simulink model "Quad_Nonlinear_Roll_Model"  (R2020a)
settings: Solver=ode4  StartTime=0.0  StopTime=0.5  FixedStep=0.01  RelTol=1e-3
values from neighbouring files (symbols this model uses):
  A1 = (h_cg * g * m_tot) / (m_tot * h_cg^2 + J_xx)    [QuadConstants.m]    (also in roll_parameter_estiation_result_I.m = 4.15251143915)
  A3 = (b * d_cg) / (m_tot * h_cg^2 + J_xx)    [QuadConstants.m]
  A5 = (m1 * g * miu_k * r_x) / (m_tot * h_cg^2 + J_xx)    [QuadConstants.m]    (also in roll_parameter_estiation_result_I.m = -0.190519012325)
  A6 = 0    [QuadConstants.m]    (also in roll_parameter_estiation_result_I.m = 0.650604724883)
  init_I = data_I(1, :)    [load_data.m]
  init_II = data_II(1, :)    [load_data.m]
  init_III = data_III(1, :)    [load_data.m]
  init_IV = data_IV(1, :)    [load_data.m]
undefined symbols (not defined in the file or in its folder): init_V, magnitude
settings Model: OrderedModelArguments=off  Creator=Ali  LastModifiedBy=Ali

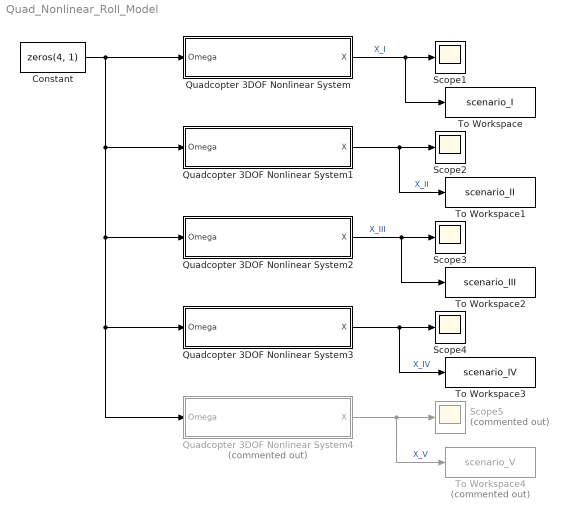
== system Quad_Nonlinear_Roll_Model ==
  Constant : Constant  Value=zeros(4, 1)
  Quadcopter 3DOF Nonlinear System : Subsystem  TreatAsAtomicUnit=on
  Quadcopter 3DOF Nonlinear System1 : Subsystem  TreatAsAtomicUnit=on
  Quadcopter 3DOF Nonlinear System2 : Subsystem  TreatAsAtomicUnit=on
  Quadcopter 3DOF Nonlinear System3 : Subsystem  TreatAsAtomicUnit=on
  Quadcopter 3DOF Nonlinear System4 : Subsystem  Commented=on  TreatAsAtomicUnit=on
  Scope{1..4} (4 alike) : Scope
  Scope5 : Scope  Commented=on
  To Workspace : ToWorkspace  VariableName=scenario_I  SampleTime=-1
  To Workspace1 : ToWorkspace  VariableName=scenario_II  SampleTime=-1
  To Workspace2 : ToWorkspace  VariableName=scenario_III  SampleTime=-1
  To Workspace3 : ToWorkspace  VariableName=scenario_IV  SampleTime=-1
  To Workspace4 : ToWorkspace  Commented=on  VariableName=scenario_V  SampleTime=-1
  wires:
  Constant/1 -> Quadcopter 3DOF Nonlinear System/1(Omega), Quadcopter 3DOF Nonlinear System4/1(Omega), Quadcopter 3DOF Nonlinear System3/1(Omega), Quadcopter 3DOF Nonlinear System2/1(Omega), Quadcopter 3DOF Nonlinear System1/1(Omega)
  Quadcopter 3DOF Nonlinear System1/1(X) -> To Workspace1/1, Scope2/1  "X_II"
  Quadcopter 3DOF Nonlinear System/1(X) -> To Workspace/1, Scope1/1  "X_I"
  Quadcopter 3DOF Nonlinear System2/1(X) -> To Workspace2/1, Scope3/1  "X_III"
  Quadcopter 3DOF Nonlinear System3/1(X) -> To Workspace3/1, Scope4/1  "X_IV"
  Quadcopter 3DOF Nonlinear System4/1(X) -> To Workspace4/1, Scope5/1  "X_V"

== system Quad_Nonlinear_Roll_Model/Quadcopter 3DOF Nonlinear System ==
  Omega : Inport
  Integrator : Integrator  InitialCondition=init_I
  Quad System : Subsystem
  X : Outport
  wires:
  Integrator/1 -> Quad System/1(X), X/1  "X"
  Quad System/1(dot(X)) -> Integrator/1  "dot(X)"
  Omega/1 -> Quad System/2(Omega)

== system Quad_Nonlinear_Roll_Model/Quadcopter 3DOF Nonlinear System1 ==
  Omega : Inport
  Integrator : Integrator  InitialCondition=init_II
  Quad System : Subsystem
  X : Outport
  wires:
  Integrator/1 -> Quad System/1(X), X/1  "X"
  Quad System/1(dot(X)) -> Integrator/1  "dot(X)"
  Omega/1 -> Quad System/2(Omega)

== system Quad_Nonlinear_Roll_Model/Quadcopter 3DOF Nonlinear System2 ==
  Omega : Inport
  Integrator : Integrator  InitialCondition=init_III
  Quad System : Subsystem
  X : Outport
  wires:
  Integrator/1 -> Quad System/1(X), X/1  "X"
  Quad System/1(dot(X)) -> Integrator/1  "dot(X)"
  Omega/1 -> Quad System/2(Omega)

== system Quad_Nonlinear_Roll_Model/Quadcopter 3DOF Nonlinear System3 ==
  Omega : Inport
  Integrator : Integrator  InitialCondition=init_IV
  Quad System : Subsystem
  X : Outport
  wires:
  Integrator/1 -> Quad System/1(X), X/1  "X"
  Quad System/1(dot(X)) -> Integrator/1  "dot(X)"
  Omega/1 -> Quad System/2(Omega)

== system Quad_Nonlinear_Roll_Model/Quadcopter 3DOF Nonlinear System4 ==
  Omega : Inport
  Integrator : Integrator  InitialCondition=init_V
  Quad System : Subsystem
  X : Outport
  wires:
  Integrator/1 -> Quad System/1(X), X/1  "X"
  Quad System/1(dot(X)) -> Integrator/1  "dot(X)"
  Omega/1 -> Quad System/2(Omega)

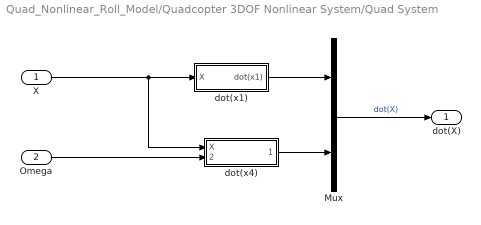
== system Quad_Nonlinear_Roll_Model/Quadcopter 3DOF Nonlinear System/Quad System ==
  X : Inport
  Omega : Inport  Port=2
  Mux : Mux  Inputs=2
  dot(x1) : Subsystem
  dot(x4) : Subsystem
  dot(X) : Outport
  wires:
  Mux/1 -> dot(X)/1  "dot(X)"
  X/1 -> dot(x4)/1(X), dot(x1)/1(X)
  Omega/1 -> dot(x4)/2(Omega)
  dot(x1)/1(dot(x1)) -> Mux/1
  dot(x4)/1(dot(x4)) -> Mux/2

== system Quad_Nonlinear_Roll_Model/Quadcopter 3DOF Nonlinear System1/Quad System ==
  X : Inport
  Omega : Inport  Port=2
  Mux : Mux  Inputs=2
  dot(x1) : Subsystem
  dot(x4) : Subsystem
  dot(X) : Outport
  wires:
  Mux/1 -> dot(X)/1  "dot(X)"
  X/1 -> dot(x4)/1(X), dot(x1)/1(X)
  Omega/1 -> dot(x4)/2(Omega)
  dot(x1)/1(dot(x1)) -> Mux/1
  dot(x4)/1(dot(x4)) -> Mux/2

== system Quad_Nonlinear_Roll_Model/Quadcopter 3DOF Nonlinear System2/Quad System ==
  X : Inport
  Omega : Inport  Port=2
  Mux : Mux  Inputs=2
  dot(x1) : Subsystem
  dot(x4) : Subsystem
  dot(X) : Outport
  wires:
  Mux/1 -> dot(X)/1  "dot(X)"
  X/1 -> dot(x4)/1(X), dot(x1)/1(X)
  Omega/1 -> dot(x4)/2(Omega)
  dot(x1)/1(dot(x1)) -> Mux/1
  dot(x4)/1(dot(x4)) -> Mux/2

== system Quad_Nonlinear_Roll_Model/Quadcopter 3DOF Nonlinear System3/Quad System ==
  X : Inport
  Omega : Inport  Port=2
  Mux : Mux  Inputs=2
  dot(x1) : Subsystem
  dot(x4) : Subsystem
  dot(X) : Outport
  wires:
  Mux/1 -> dot(X)/1  "dot(X)"
  X/1 -> dot(x4)/1(X), dot(x1)/1(X)
  Omega/1 -> dot(x4)/2(Omega)
  dot(x1)/1(dot(x1)) -> Mux/1
  dot(x4)/1(dot(x4)) -> Mux/2

== system Quad_Nonlinear_Roll_Model/Quadcopter 3DOF Nonlinear System4/Quad System ==
  X : Inport
  Omega : Inport  Port=2
  Mux : Mux  Inputs=2
  dot(x1) : Subsystem
  dot(x4) : Subsystem
  dot(X) : Outport
  wires:
  Mux/1 -> dot(X)/1  "dot(X)"
  X/1 -> dot(x4)/1(X), dot(x1)/1(X)
  Omega/1 -> dot(x4)/2(Omega)
  dot(x1)/1(dot(x1)) -> Mux/1
  dot(x4)/1(dot(x4)) -> Mux/2

== system Quad_Nonlinear_Roll_Model/Quadcopter 3DOF Nonlinear System/Quad System/dot(x1) ==
  X : Inport
  Subsystem1 : Subsystem
  dot(x1) : Outport
  wires:
  X/1 -> Subsystem1/1(X)  "X"
  Subsystem1/1(x4) -> dot(x1)/1

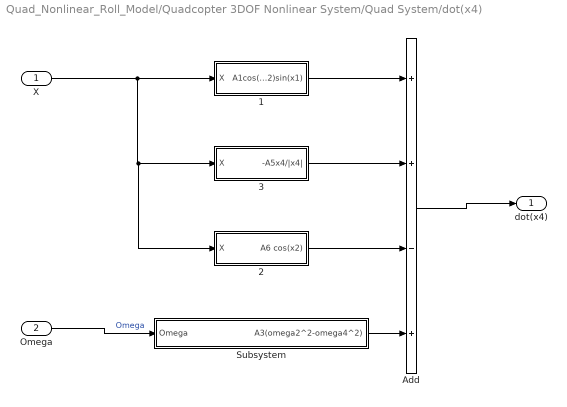
== system Quad_Nonlinear_Roll_Model/Quadcopter 3DOF Nonlinear System/Quad System/dot(x4) ==
  X : Inport
  Omega : Inport  Port=2
  1 : Subsystem
  2 : Subsystem
  3 : Subsystem
  Add : Sum  Inputs=++-+
  Subsystem : Subsystem
  dot(x4) : Outport
  wires:
  Omega/1 -> Subsystem/1(Omega)  "Omega"
  Add/1 -> dot(x4)/1
  1/1(A1cos(x2)sin(x1)) -> Add/1
  3/1("-A5x4/|x4| ") -> Add/2
  X/1 -> 2/1(X), 3/1(X), 1/1(X)
  2/1(A6 cos(x2)) -> Add/3
  Subsystem/1(A3(omega2^2-omega4^2)) -> Add/4

== system Quad_Nonlinear_Roll_Model/Quadcopter 3DOF Nonlinear System1/Quad System/dot(x1) ==
  X : Inport
  Subsystem1 : Subsystem
  dot(x1) : Outport
  wires:
  X/1 -> Subsystem1/1(X)  "X"
  Subsystem1/1(x4) -> dot(x1)/1

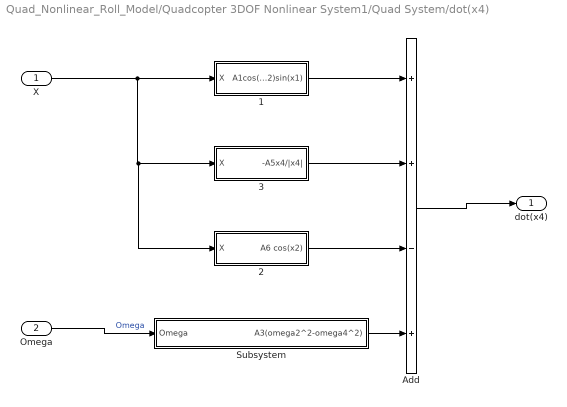
== system Quad_Nonlinear_Roll_Model/Quadcopter 3DOF Nonlinear System1/Quad System/dot(x4) ==
  X : Inport
  Omega : Inport  Port=2
  1 : Subsystem
  2 : Subsystem
  3 : Subsystem
  Add : Sum  Inputs=++-+
  Subsystem : Subsystem
  dot(x4) : Outport
  wires:
  Omega/1 -> Subsystem/1(Omega)  "Omega"
  Add/1 -> dot(x4)/1
  1/1(A1cos(x2)sin(x1)) -> Add/1
  3/1("-A5x4/|x4| ") -> Add/2
  X/1 -> 2/1(X), 3/1(X), 1/1(X)
  2/1(A6 cos(x2)) -> Add/3
  Subsystem/1(A3(omega2^2-omega4^2)) -> Add/4

== system Quad_Nonlinear_Roll_Model/Quadcopter 3DOF Nonlinear System2/Quad System/dot(x1) ==
  X : Inport
  Subsystem1 : Subsystem
  dot(x1) : Outport
  wires:
  X/1 -> Subsystem1/1(X)  "X"
  Subsystem1/1(x4) -> dot(x1)/1

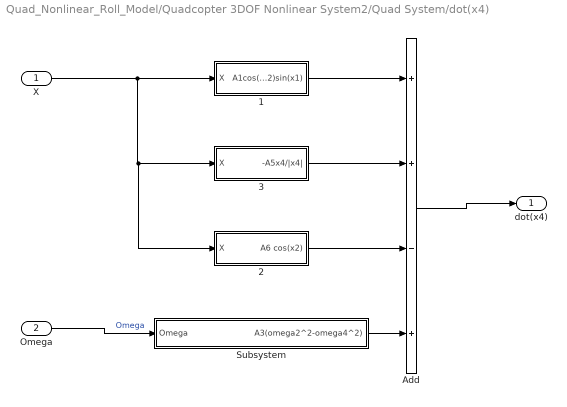
== system Quad_Nonlinear_Roll_Model/Quadcopter 3DOF Nonlinear System2/Quad System/dot(x4) ==
  X : Inport
  Omega : Inport  Port=2
  1 : Subsystem
  2 : Subsystem
  3 : Subsystem
  Add : Sum  Inputs=++-+
  Subsystem : Subsystem
  dot(x4) : Outport
  wires:
  Omega/1 -> Subsystem/1(Omega)  "Omega"
  Add/1 -> dot(x4)/1
  1/1(A1cos(x2)sin(x1)) -> Add/1
  3/1("-A5x4/|x4| ") -> Add/2
  X/1 -> 2/1(X), 3/1(X), 1/1(X)
  2/1(A6 cos(x2)) -> Add/3
  Subsystem/1(A3(omega2^2-omega4^2)) -> Add/4

== system Quad_Nonlinear_Roll_Model/Quadcopter 3DOF Nonlinear System3/Quad System/dot(x1) ==
  X : Inport
  Subsystem1 : Subsystem
  dot(x1) : Outport
  wires:
  X/1 -> Subsystem1/1(X)  "X"
  Subsystem1/1(x4) -> dot(x1)/1

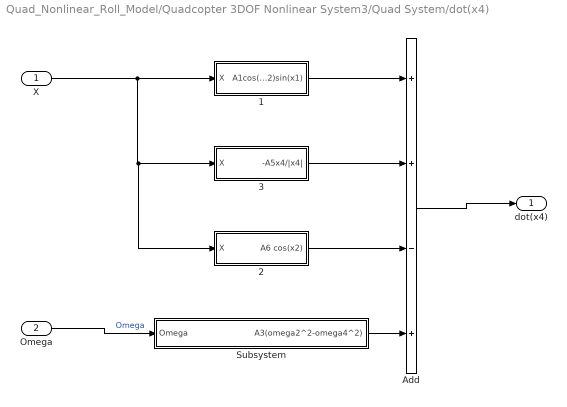
== system Quad_Nonlinear_Roll_Model/Quadcopter 3DOF Nonlinear System3/Quad System/dot(x4) ==
  X : Inport
  Omega : Inport  Port=2
  1 : Subsystem
  2 : Subsystem
  3 : Subsystem
  Add : Sum  Inputs=++-+
  Subsystem : Subsystem
  dot(x4) : Outport
  wires:
  Omega/1 -> Subsystem/1(Omega)  "Omega"
  Add/1 -> dot(x4)/1
  1/1(A1cos(x2)sin(x1)) -> Add/1
  3/1("-A5x4/|x4| ") -> Add/2
  X/1 -> 2/1(X), 3/1(X), 1/1(X)
  2/1(A6 cos(x2)) -> Add/3
  Subsystem/1(A3(omega2^2-omega4^2)) -> Add/4

== system Quad_Nonlinear_Roll_Model/Quadcopter 3DOF Nonlinear System4/Quad System/dot(x1) ==
  X : Inport
  Subsystem1 : Subsystem
  dot(x1) : Outport
  wires:
  X/1 -> Subsystem1/1(X)  "X"
  Subsystem1/1(x4) -> dot(x1)/1

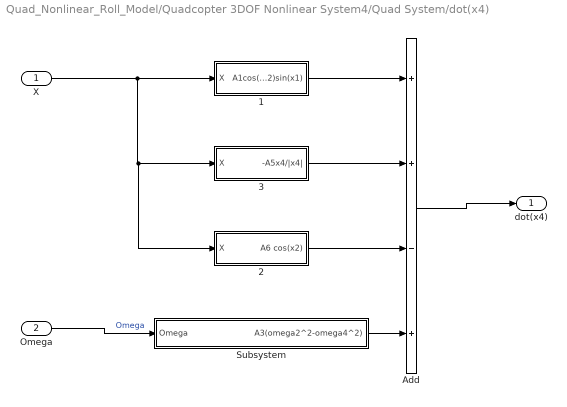
== system Quad_Nonlinear_Roll_Model/Quadcopter 3DOF Nonlinear System4/Quad System/dot(x4) ==
  X : Inport
  Omega : Inport  Port=2
  1 : Subsystem
  2 : Subsystem
  3 : Subsystem
  Add : Sum  Inputs=++-+
  Subsystem : Subsystem
  dot(x4) : Outport
  wires:
  Omega/1 -> Subsystem/1(Omega)  "Omega"
  Add/1 -> dot(x4)/1
  1/1(A1cos(x2)sin(x1)) -> Add/1
  3/1("-A5x4/|x4| ") -> Add/2
  X/1 -> 2/1(X), 3/1(X), 1/1(X)
  2/1(A6 cos(x2)) -> Add/3
  Subsystem/1(A3(omega2^2-omega4^2)) -> Add/4

== system Quad_Nonlinear_Roll_Model/Quadcopter 3DOF Nonlinear System/Quad System/dot(x1)/Subsystem1 ==
  X : Inport
  Selector : Selector  InputPortWidth=2  IndexOptions=Index vector (dialog)  Indices=[2]  OutputSizes=1
  x4 : Outport
  wires:
  Selector/1 -> x4/1
  X/1 -> Selector/1

== system Quad_Nonlinear_Roll_Model/Quadcopter 3DOF Nonlinear System/Quad System/dot(x4)/1 ==
  X : Inport
  Selector : Selector  InputPortWidth=2  IndexOptions=Index vector (dialog)  Indices=[1]  OutputSizes=1
  Subsystem : Subsystem
  A1cos(x2)sin(x1) : Outport
  wires:
  Selector/1 -> Subsystem/1(x1)  "x1"
  Subsystem/1(A1cos(x2)sin(x1)) -> A1cos(x2)sin(x1)/1
  X/1 -> Selector/1  "x"

== system Quad_Nonlinear_Roll_Model/Quadcopter 3DOF Nonlinear System/Quad System/dot(x4)/2 ==
  X : Inport
  Selector : Selector  InputPortWidth=2  IndexOptions=Index vector (dialog)  Indices=[1]  OutputSizes=1
  Subsystem : Subsystem
  A6 cos(x2) : Outport
  wires:
  X/1 -> Selector/1  "x"
  Subsystem/1(A6 cos(x1)) -> A6 cos(x2)/1
  Selector/1 -> Subsystem/1(x1)

== system Quad_Nonlinear_Roll_Model/Quadcopter 3DOF Nonlinear System/Quad System/dot(x4)/3 ==
  X : Inport
  Selector : Selector  InputPortWidth=2  IndexOptions=Index vector (dialog)  Indices=[2]  OutputSizes=1
  Subsystem : Subsystem
  "-A5x4/|x4| " : Outport
  wires:
  Subsystem/1("-A5x4/|x4| ") -> "-A5x4/|x4| "/1
  X/1 -> Selector/1  "x"
  Selector/1 -> Subsystem/1(x4)

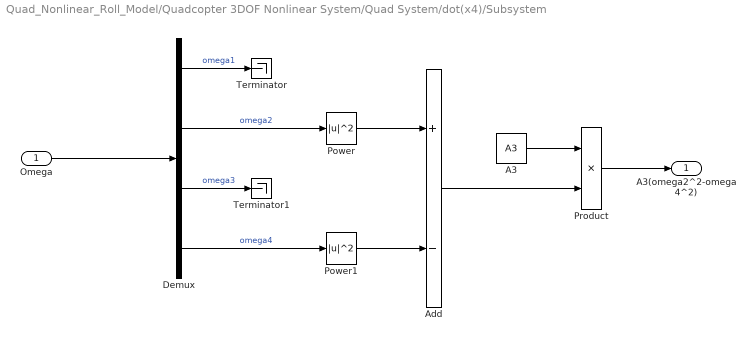
== system Quad_Nonlinear_Roll_Model/Quadcopter 3DOF Nonlinear System/Quad System/dot(x4)/Subsystem ==
  Omega : Inport
  A3 : Constant  Value=A3
  Add : Sum  Inputs=+-
  Demux : Demux
  Power : Math  Operator=magnitude^2  SaturateOnIntegerOverflow=on
  Power1 : Math  Operator=magnitude^2  SaturateOnIntegerOverflow=on
  Product : Product
  Terminator : Terminator
  Terminator1 : Terminator
  A3(omega2^2-omega4^2) : Outport
  wires:
  Product/1 -> A3(omega2^2-omega4^2)/1
  Power1/1 -> Add/2
  Demux/2 -> Power/1  "omega2"
  Demux/4 -> Power1/1  "omega4"
  Add/1 -> Product/2
  Power/1 -> Add/1
  A3/1 -> Product/1
  Omega/1 -> Demux/1
  Demux/3 -> Terminator1/1  "omega3"
  Demux/1 -> Terminator/1  "omega1"

== system Quad_Nonlinear_Roll_Model/Quadcopter 3DOF Nonlinear System1/Quad System/dot(x1)/Subsystem1 ==
  X : Inport
  Selector : Selector  InputPortWidth=2  IndexOptions=Index vector (dialog)  Indices=[2]  OutputSizes=1
  x4 : Outport
  wires:
  Selector/1 -> x4/1
  X/1 -> Selector/1

== system Quad_Nonlinear_Roll_Model/Quadcopter 3DOF Nonlinear System1/Quad System/dot(x4)/1 ==
  X : Inport
  Selector : Selector  InputPortWidth=2  IndexOptions=Index vector (dialog)  Indices=[1]  OutputSizes=1
  Subsystem : Subsystem
  A1cos(x2)sin(x1) : Outport
  wires:
  Selector/1 -> Subsystem/1(x1)  "x1"
  Subsystem/1(A1cos(x2)sin(x1)) -> A1cos(x2)sin(x1)/1
  X/1 -> Selector/1  "x"

== system Quad_Nonlinear_Roll_Model/Quadcopter 3DOF Nonlinear System1/Quad System/dot(x4)/2 ==
  X : Inport
  Selector : Selector  InputPortWidth=2  IndexOptions=Index vector (dialog)  Indices=[1]  OutputSizes=1
  Subsystem : Subsystem
  A6 cos(x2) : Outport
  wires:
  X/1 -> Selector/1  "x"
  Subsystem/1(A6 cos(x1)) -> A6 cos(x2)/1
  Selector/1 -> Subsystem/1(x1)

== system Quad_Nonlinear_Roll_Model/Quadcopter 3DOF Nonlinear System1/Quad System/dot(x4)/3 ==
  X : Inport
  Selector : Selector  InputPortWidth=2  IndexOptions=Index vector (dialog)  Indices=[2]  OutputSizes=1
  Subsystem : Subsystem
  "-A5x4/|x4| " : Outport
  wires:
  Subsystem/1("-A5x4/|x4| ") -> "-A5x4/|x4| "/1
  X/1 -> Selector/1  "x"
  Selector/1 -> Subsystem/1(x4)

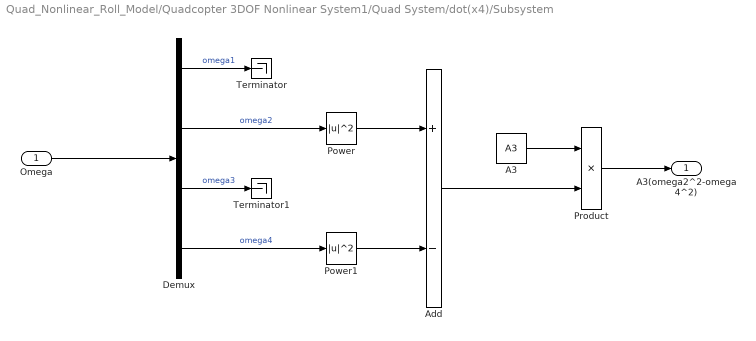
== system Quad_Nonlinear_Roll_Model/Quadcopter 3DOF Nonlinear System1/Quad System/dot(x4)/Subsystem ==
  Omega : Inport
  A3 : Constant  Value=A3
  Add : Sum  Inputs=+-
  Demux : Demux
  Power : Math  Operator=magnitude^2  SaturateOnIntegerOverflow=on
  Power1 : Math  Operator=magnitude^2  SaturateOnIntegerOverflow=on
  Product : Product
  Terminator : Terminator
  Terminator1 : Terminator
  A3(omega2^2-omega4^2) : Outport
  wires:
  Product/1 -> A3(omega2^2-omega4^2)/1
  Power1/1 -> Add/2
  Demux/2 -> Power/1  "omega2"
  Demux/4 -> Power1/1  "omega4"
  Add/1 -> Product/2
  Power/1 -> Add/1
  A3/1 -> Product/1
  Omega/1 -> Demux/1
  Demux/3 -> Terminator1/1  "omega3"
  Demux/1 -> Terminator/1  "omega1"

== system Quad_Nonlinear_Roll_Model/Quadcopter 3DOF Nonlinear System2/Quad System/dot(x1)/Subsystem1 ==
  X : Inport
  Selector : Selector  InputPortWidth=2  IndexOptions=Index vector (dialog)  Indices=[2]  OutputSizes=1
  x4 : Outport
  wires:
  Selector/1 -> x4/1
  X/1 -> Selector/1

== system Quad_Nonlinear_Roll_Model/Quadcopter 3DOF Nonlinear System2/Quad System/dot(x4)/1 ==
  X : Inport
  Selector : Selector  InputPortWidth=2  IndexOptions=Index vector (dialog)  Indices=[1]  OutputSizes=1
  Subsystem : Subsystem
  A1cos(x2)sin(x1) : Outport
  wires:
  Selector/1 -> Subsystem/1(x1)  "x1"
  Subsystem/1(A1cos(x2)sin(x1)) -> A1cos(x2)sin(x1)/1
  X/1 -> Selector/1  "x"

== system Quad_Nonlinear_Roll_Model/Quadcopter 3DOF Nonlinear System2/Quad System/dot(x4)/2 ==
  X : Inport
  Selector : Selector  InputPortWidth=2  IndexOptions=Index vector (dialog)  Indices=[1]  OutputSizes=1
  Subsystem : Subsystem
  A6 cos(x2) : Outport
  wires:
  X/1 -> Selector/1  "x"
  Subsystem/1(A6 cos(x1)) -> A6 cos(x2)/1
  Selector/1 -> Subsystem/1(x1)

== system Quad_Nonlinear_Roll_Model/Quadcopter 3DOF Nonlinear System2/Quad System/dot(x4)/3 ==
  X : Inport
  Selector : Selector  InputPortWidth=2  IndexOptions=Index vector (dialog)  Indices=[2]  OutputSizes=1
  Subsystem : Subsystem
  "-A5x4/|x4| " : Outport
  wires:
  Subsystem/1("-A5x4/|x4| ") -> "-A5x4/|x4| "/1
  X/1 -> Selector/1  "x"
  Selector/1 -> Subsystem/1(x4)

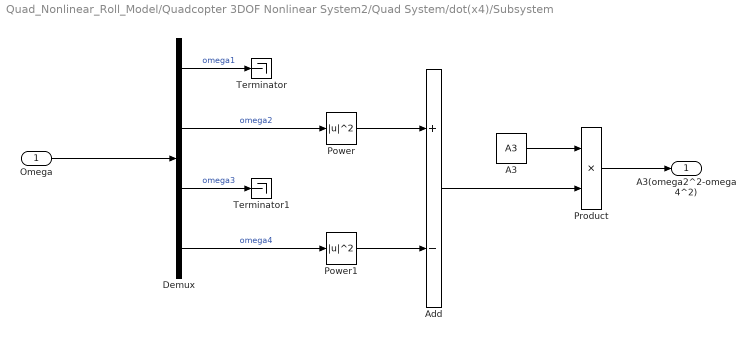
== system Quad_Nonlinear_Roll_Model/Quadcopter 3DOF Nonlinear System2/Quad System/dot(x4)/Subsystem ==
  Omega : Inport
  A3 : Constant  Value=A3
  Add : Sum  Inputs=+-
  Demux : Demux
  Power : Math  Operator=magnitude^2  SaturateOnIntegerOverflow=on
  Power1 : Math  Operator=magnitude^2  SaturateOnIntegerOverflow=on
  Product : Product
  Terminator : Terminator
  Terminator1 : Terminator
  A3(omega2^2-omega4^2) : Outport
  wires:
  Product/1 -> A3(omega2^2-omega4^2)/1
  Power1/1 -> Add/2
  Demux/2 -> Power/1  "omega2"
  Demux/4 -> Power1/1  "omega4"
  Add/1 -> Product/2
  Power/1 -> Add/1
  A3/1 -> Product/1
  Omega/1 -> Demux/1
  Demux/3 -> Terminator1/1  "omega3"
  Demux/1 -> Terminator/1  "omega1"

== system Quad_Nonlinear_Roll_Model/Quadcopter 3DOF Nonlinear System3/Quad System/dot(x1)/Subsystem1 ==
  X : Inport
  Selector : Selector  InputPortWidth=2  IndexOptions=Index vector (dialog)  Indices=[2]  OutputSizes=1
  x4 : Outport
  wires:
  Selector/1 -> x4/1
  X/1 -> Selector/1

== system Quad_Nonlinear_Roll_Model/Quadcopter 3DOF Nonlinear System3/Quad System/dot(x4)/1 ==
  X : Inport
  Selector : Selector  InputPortWidth=2  IndexOptions=Index vector (dialog)  Indices=[1]  OutputSizes=1
  Subsystem : Subsystem
  A1cos(x2)sin(x1) : Outport
  wires:
  Selector/1 -> Subsystem/1(x1)  "x1"
  Subsystem/1(A1cos(x2)sin(x1)) -> A1cos(x2)sin(x1)/1
  X/1 -> Selector/1  "x"

== system Quad_Nonlinear_Roll_Model/Quadcopter 3DOF Nonlinear System3/Quad System/dot(x4)/2 ==
  X : Inport
  Selector : Selector  InputPortWidth=2  IndexOptions=Index vector (dialog)  Indices=[1]  OutputSizes=1
  Subsystem : Subsystem
  A6 cos(x2) : Outport
  wires:
  X/1 -> Selector/1  "x"
  Subsystem/1(A6 cos(x1)) -> A6 cos(x2)/1
  Selector/1 -> Subsystem/1(x1)

== system Quad_Nonlinear_Roll_Model/Quadcopter 3DOF Nonlinear System3/Quad System/dot(x4)/3 ==
  X : Inport
  Selector : Selector  InputPortWidth=2  IndexOptions=Index vector (dialog)  Indices=[2]  OutputSizes=1
  Subsystem : Subsystem
  "-A5x4/|x4| " : Outport
  wires:
  Subsystem/1("-A5x4/|x4| ") -> "-A5x4/|x4| "/1
  X/1 -> Selector/1  "x"
  Selector/1 -> Subsystem/1(x4)

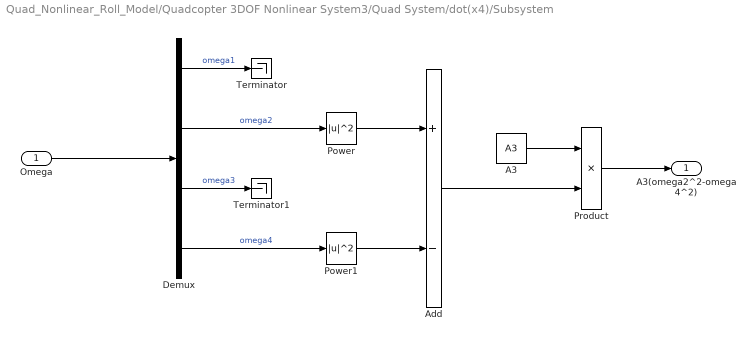
== system Quad_Nonlinear_Roll_Model/Quadcopter 3DOF Nonlinear System3/Quad System/dot(x4)/Subsystem ==
  Omega : Inport
  A3 : Constant  Value=A3
  Add : Sum  Inputs=+-
  Demux : Demux
  Power : Math  Operator=magnitude^2  SaturateOnIntegerOverflow=on
  Power1 : Math  Operator=magnitude^2  SaturateOnIntegerOverflow=on
  Product : Product
  Terminator : Terminator
  Terminator1 : Terminator
  A3(omega2^2-omega4^2) : Outport
  wires:
  Product/1 -> A3(omega2^2-omega4^2)/1
  Power1/1 -> Add/2
  Demux/2 -> Power/1  "omega2"
  Demux/4 -> Power1/1  "omega4"
  Add/1 -> Product/2
  Power/1 -> Add/1
  A3/1 -> Product/1
  Omega/1 -> Demux/1
  Demux/3 -> Terminator1/1  "omega3"
  Demux/1 -> Terminator/1  "omega1"

== system Quad_Nonlinear_Roll_Model/Quadcopter 3DOF Nonlinear System4/Quad System/dot(x1)/Subsystem1 ==
  X : Inport
  Selector : Selector  InputPortWidth=2  IndexOptions=Index vector (dialog)  Indices=[2]  OutputSizes=1
  x4 : Outport
  wires:
  Selector/1 -> x4/1
  X/1 -> Selector/1

== system Quad_Nonlinear_Roll_Model/Quadcopter 3DOF Nonlinear System4/Quad System/dot(x4)/1 ==
  X : Inport
  Selector : Selector  InputPortWidth=2  IndexOptions=Index vector (dialog)  Indices=[1]  OutputSizes=1
  Subsystem : Subsystem
  A1cos(x2)sin(x1) : Outport
  wires:
  Selector/1 -> Subsystem/1(x1)  "x1"
  Subsystem/1(A1cos(x2)sin(x1)) -> A1cos(x2)sin(x1)/1
  X/1 -> Selector/1  "x"

== system Quad_Nonlinear_Roll_Model/Quadcopter 3DOF Nonlinear System4/Quad System/dot(x4)/2 ==
  X : Inport
  Selector : Selector  InputPortWidth=2  IndexOptions=Index vector (dialog)  Indices=[1]  OutputSizes=1
  Subsystem : Subsystem
  A6 cos(x2) : Outport
  wires:
  X/1 -> Selector/1  "x"
  Subsystem/1(A6 cos(x1)) -> A6 cos(x2)/1
  Selector/1 -> Subsystem/1(x1)

== system Quad_Nonlinear_Roll_Model/Quadcopter 3DOF Nonlinear System4/Quad System/dot(x4)/3 ==
  X : Inport
  Selector : Selector  InputPortWidth=2  IndexOptions=Index vector (dialog)  Indices=[2]  OutputSizes=1
  Subsystem : Subsystem
  "-A5x4/|x4| " : Outport
  wires:
  Subsystem/1("-A5x4/|x4| ") -> "-A5x4/|x4| "/1
  X/1 -> Selector/1  "x"
  Selector/1 -> Subsystem/1(x4)

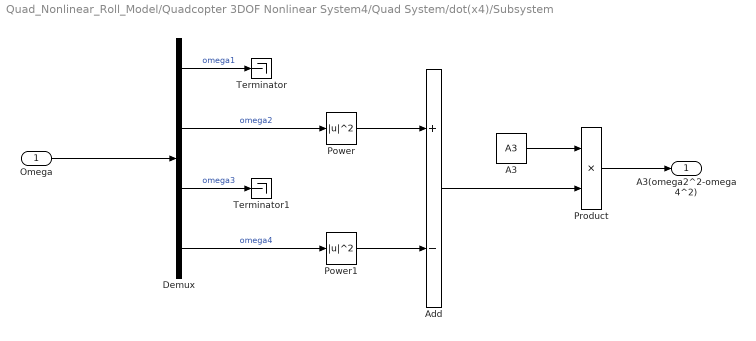
== system Quad_Nonlinear_Roll_Model/Quadcopter 3DOF Nonlinear System4/Quad System/dot(x4)/Subsystem ==
  Omega : Inport
  A3 : Constant  Value=A3
  Add : Sum  Inputs=+-
  Demux : Demux
  Power : Math  Operator=magnitude^2  SaturateOnIntegerOverflow=on
  Power1 : Math  Operator=magnitude^2  SaturateOnIntegerOverflow=on
  Product : Product
  Terminator : Terminator
  Terminator1 : Terminator
  A3(omega2^2-omega4^2) : Outport
  wires:
  Product/1 -> A3(omega2^2-omega4^2)/1
  Power1/1 -> Add/2
  Demux/2 -> Power/1  "omega2"
  Demux/4 -> Power1/1  "omega4"
  Add/1 -> Product/2
  Power/1 -> Add/1
  A3/1 -> Product/1
  Omega/1 -> Demux/1
  Demux/3 -> Terminator1/1  "omega3"
  Demux/1 -> Terminator/1  "omega1"

== system Quad_Nonlinear_Roll_Model/Quadcopter 3DOF Nonlinear System/Quad System/dot(x4)/1/Subsystem ==
  x1 : Inport
  A1 : Constant  Value=A1
  Product : Product
  Sin : Trigonometry
  A1cos(x2)sin(x1) : Outport
  wires:
  Sin/1 -> Product/1
  Product/1 -> A1cos(x2)sin(x1)/1
  x1/1 -> Sin/1
  A1/1 -> Product/2

== system Quad_Nonlinear_Roll_Model/Quadcopter 3DOF Nonlinear System/Quad System/dot(x4)/2/Subsystem ==
  x1 : Inport
  A6 : Constant  Value=A6
  Cos : Trigonometry  Operator=cos
  Product : Product
  A6 cos(x1) : Outport
  wires:
  A6/1 -> Product/1
  Product/1 -> A6 cos(x1)/1
  x1/1 -> Cos/1
  Cos/1 -> Product/2

== system Quad_Nonlinear_Roll_Model/Quadcopter 3DOF Nonlinear System/Quad System/dot(x4)/3/Subsystem ==
  x4 : Inport
  A5 : Constant  Value=A5
  Gain : Gain  Gain=-1
  Switch : Switch  Criteria=u2 > Threshold
  "-A5x4/|x4| " : Outport
  wires:
  Switch/1 -> "-A5x4/|x4| "/1
  A5/1 -> Switch/3, Gain/1
  x4/1 -> Switch/2
  Gain/1 -> Switch/1

== system Quad_Nonlinear_Roll_Model/Quadcopter 3DOF Nonlinear System1/Quad System/dot(x4)/1/Subsystem ==
  x1 : Inport
  A1 : Constant  Value=A1
  Product : Product
  Sin : Trigonometry
  A1cos(x2)sin(x1) : Outport
  wires:
  Sin/1 -> Product/1
  Product/1 -> A1cos(x2)sin(x1)/1
  x1/1 -> Sin/1
  A1/1 -> Product/2

== system Quad_Nonlinear_Roll_Model/Quadcopter 3DOF Nonlinear System1/Quad System/dot(x4)/2/Subsystem ==
  x1 : Inport
  A6 : Constant  Value=A6
  Cos : Trigonometry  Operator=cos
  Product : Product
  A6 cos(x1) : Outport
  wires:
  A6/1 -> Product/1
  Product/1 -> A6 cos(x1)/1
  x1/1 -> Cos/1
  Cos/1 -> Product/2

== system Quad_Nonlinear_Roll_Model/Quadcopter 3DOF Nonlinear System1/Quad System/dot(x4)/3/Subsystem ==
  x4 : Inport
  A5 : Constant  Value=A5
  Gain : Gain  Gain=-1
  Switch : Switch  Criteria=u2 > Threshold
  "-A5x4/|x4| " : Outport
  wires:
  Switch/1 -> "-A5x4/|x4| "/1
  A5/1 -> Switch/3, Gain/1
  x4/1 -> Switch/2
  Gain/1 -> Switch/1

== system Quad_Nonlinear_Roll_Model/Quadcopter 3DOF Nonlinear System2/Quad System/dot(x4)/1/Subsystem ==
  x1 : Inport
  A1 : Constant  Value=A1
  Product : Product
  Sin : Trigonometry
  A1cos(x2)sin(x1) : Outport
  wires:
  Sin/1 -> Product/1
  Product/1 -> A1cos(x2)sin(x1)/1
  x1/1 -> Sin/1
  A1/1 -> Product/2

== system Quad_Nonlinear_Roll_Model/Quadcopter 3DOF Nonlinear System2/Quad System/dot(x4)/2/Subsystem ==
  x1 : Inport
  A6 : Constant  Value=A6
  Cos : Trigonometry  Operator=cos
  Product : Product
  A6 cos(x1) : Outport
  wires:
  A6/1 -> Product/1
  Product/1 -> A6 cos(x1)/1
  x1/1 -> Cos/1
  Cos/1 -> Product/2

== system Quad_Nonlinear_Roll_Model/Quadcopter 3DOF Nonlinear System2/Quad System/dot(x4)/3/Subsystem ==
  x4 : Inport
  A5 : Constant  Value=A5
  Gain : Gain  Gain=-1
  Switch : Switch  Criteria=u2 > Threshold
  "-A5x4/|x4| " : Outport
  wires:
  Switch/1 -> "-A5x4/|x4| "/1
  A5/1 -> Switch/3, Gain/1
  x4/1 -> Switch/2
  Gain/1 -> Switch/1

== system Quad_Nonlinear_Roll_Model/Quadcopter 3DOF Nonlinear System3/Quad System/dot(x4)/1/Subsystem ==
  x1 : Inport
  A1 : Constant  Value=A1
  Product : Product
  Sin : Trigonometry
  A1cos(x2)sin(x1) : Outport
  wires:
  Sin/1 -> Product/1
  Product/1 -> A1cos(x2)sin(x1)/1
  x1/1 -> Sin/1
  A1/1 -> Product/2

== system Quad_Nonlinear_Roll_Model/Quadcopter 3DOF Nonlinear System3/Quad System/dot(x4)/2/Subsystem ==
  x1 : Inport
  A6 : Constant  Value=A6
  Cos : Trigonometry  Operator=cos
  Product : Product
  A6 cos(x1) : Outport
  wires:
  A6/1 -> Product/1
  Product/1 -> A6 cos(x1)/1
  x1/1 -> Cos/1
  Cos/1 -> Product/2

== system Quad_Nonlinear_Roll_Model/Quadcopter 3DOF Nonlinear System3/Quad System/dot(x4)/3/Subsystem ==
  x4 : Inport
  A5 : Constant  Value=A5
  Gain : Gain  Gain=-1
  Switch : Switch  Criteria=u2 > Threshold
  "-A5x4/|x4| " : Outport
  wires:
  Switch/1 -> "-A5x4/|x4| "/1
  A5/1 -> Switch/3, Gain/1
  x4/1 -> Switch/2
  Gain/1 -> Switch/1

== system Quad_Nonlinear_Roll_Model/Quadcopter 3DOF Nonlinear System4/Quad System/dot(x4)/1/Subsystem ==
  x1 : Inport
  A1 : Constant  Value=A1
  Product : Product
  Sin : Trigonometry
  A1cos(x2)sin(x1) : Outport
  wires:
  Sin/1 -> Product/1
  Product/1 -> A1cos(x2)sin(x1)/1
  x1/1 -> Sin/1
  A1/1 -> Product/2

== system Quad_Nonlinear_Roll_Model/Quadcopter 3DOF Nonlinear System4/Quad System/dot(x4)/2/Subsystem ==
  x1 : Inport
  A6 : Constant  Value=A6
  Cos : Trigonometry  Operator=cos
  Product : Product
  A6 cos(x1) : Outport
  wires:
  A6/1 -> Product/1
  Product/1 -> A6 cos(x1)/1
  x1/1 -> Cos/1
  Cos/1 -> Product/2

== system Quad_Nonlinear_Roll_Model/Quadcopter 3DOF Nonlinear System4/Quad System/dot(x4)/3/Subsystem ==
  x4 : Inport
  A5 : Constant  Value=A5
  Gain : Gain  Gain=-1
  Switch : Switch  Criteria=u2 > Threshold
  "-A5x4/|x4| " : Outport
  wires:
  Switch/1 -> "-A5x4/|x4| "/1
  A5/1 -> Switch/3, Gain/1
  x4/1 -> Switch/2
  Gain/1 -> Switch/1
